simulink model "Roadsense_BehaviourPlanner"  (R2025b)
settings: Solver=FixedStepDiscrete  StartTime=0.0  StopTime=1.0  FixedStep=RsTsBase  RelTol=1e-3
undefined symbols (not defined in the file or in its folder): RsBehaviourEmergencyHoldTicks, RsBehaviourYieldClearTicks, RsGridCols, RsGridRows, RsMaxTracks, RsTsPlanning
settings Model: DataDictionary=Roadsense_Data.sldd  Creator=ragur  LastModifiedBy=ragur

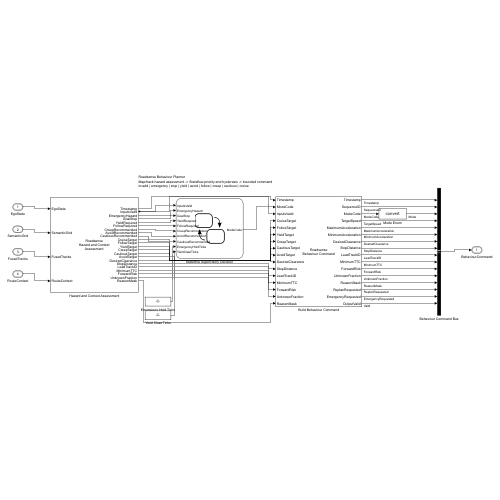
[thumbnail: Simulink's stored preview of the top-level diagram]
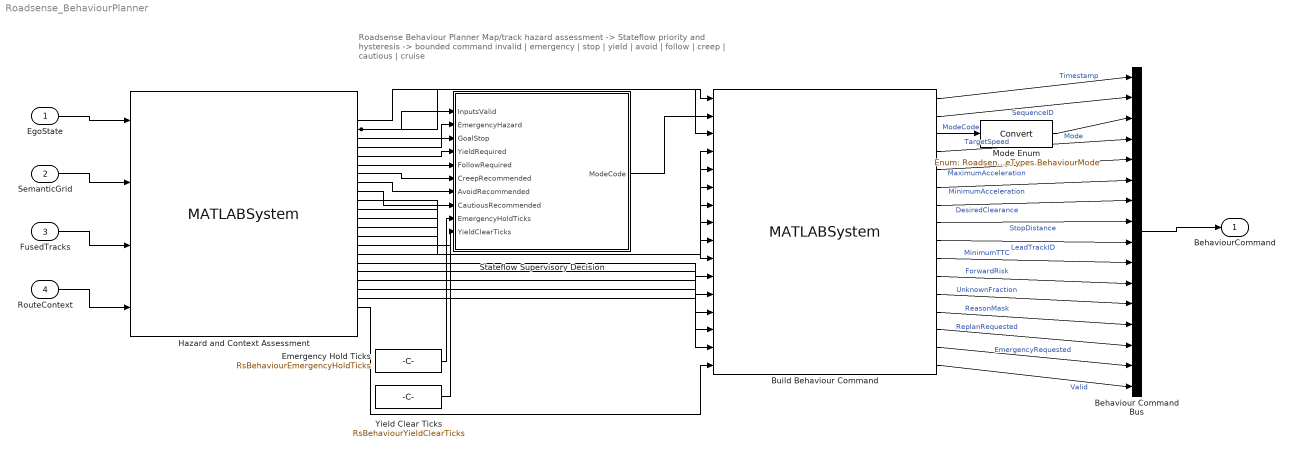
== system Roadsense_BehaviourPlanner ==
  note: Roadsense Behaviour Planner
      | Map/track hazard assessment -> Stateflow priority and hysteresis -> bounded command
      | invalid | emergency | stop | yield | avoid | follow | creep | cautious | cruise
  EgoState : Inport  OutDataTypeStr=Bus: RsEgoStateBus  PortDimensions=1  SampleTime=RsTsPlanning
  SemanticGrid : Inport  Port=2  OutDataTypeStr=Bus: RsSemanticGridBus  PortDimensions=1  SampleTime=RsTsPlanning
  FusedTracks : Inport  Port=3  OutDataTypeStr=Bus: RsFusedTrackListBus  PortDimensions=1  SampleTime=RsTsPlanning
  RouteContext : Inport  Port=4  OutDataTypeStr=Bus: RsRouteContextBus  PortDimensions=1  SampleTime=RsTsPlanning
  Behaviour Command Bus : BusCreator  Inputs=16  OutDataTypeStr=Bus: RsBehaviourCommandBus
  Build Behaviour Command : MATLABSystem  System=RoadsenseBehaviourCommandSystem  SimulateUsing=Code generation
      mask Type: RoadsenseBehaviourCommandSystem
  Emergency Hold Ticks : Constant  Value=RsBehaviourEmergencyHoldTicks  OutDataTypeStr=uint16
  Hazard and Context Assessment : MATLABSystem  System=RoadsenseBehaviourAssessmentSystem  MaxTracks=double(RsMaxTracks)  GridRows=double(RsGridRows)  GridCols=double(RsGridCols)  GridResolution=RsGridResolution  GridXLimits=RsGridXLimits  GridYLimits=RsGridYLimits  ReactionTime=RsBehaviourReactionTime  EmergencyDeceleration=RsBehaviourEmergencyDeceleration  ComfortDeceleration=RsBehaviourComfortDeceleration  EmergencyTTC=RsBehaviourEmergencyTTC  FollowTimeGap=RsBehaviourFollowTimeGap  CreepSpeed=RsBehaviourCreepSpeed  CautiousSpeed=RsBehaviourCautiousSpeed  AvoidSpeed=RsBehaviourAvoidSpeed  SimulateUsing=Code generation
      mask Type: RoadsenseBehaviourAssessmentSystem
  Mode Enum : DataTypeConversion  OutDataTypeStr=Enum: RoadsenseTypes.BehaviourMode  SaturateOnIntegerOverflow=off  RndMeth=Floor
  Stateflow Supervisory Decision : Stateflow chart  TreatAsAtomicUnit=on
  Yield Clear Ticks : Constant  Value=RsBehaviourYieldClearTicks  OutDataTypeStr=uint16
  BehaviourCommand : Outport  OutDataTypeStr=Bus: RsBehaviourCommandBus
  wires:
  EgoState/1 -> Hazard and Context Assessment/1
  SemanticGrid/1 -> Hazard and Context Assessment/2
  FusedTracks/1 -> Hazard and Context Assessment/3
  RouteContext/1 -> Hazard and Context Assessment/4
  Hazard and Context Assessment/2 -> Stateflow Supervisory Decision/1(InputsValid), Build Behaviour Command/3
  Hazard and Context Assessment/3 -> Stateflow Supervisory Decision/2(EmergencyHazard)
  Hazard and Context Assessment/4 -> Stateflow Supervisory Decision/3(GoalStop)
  Hazard and Context Assessment/5 -> Stateflow Supervisory Decision/4(YieldRequired)
  Hazard and Context Assessment/6 -> Stateflow Supervisory Decision/5(FollowRequired)
  Hazard and Context Assessment/7 -> Stateflow Supervisory Decision/6(CreepRecommended)
  Hazard and Context Assessment/8 -> Stateflow Supervisory Decision/7(AvoidRecommended)
  Hazard and Context Assessment/9 -> Stateflow Supervisory Decision/8(CautiousRecommended)
  Emergency Hold Ticks/1 -> Stateflow Supervisory Decision/9(EmergencyHoldTicks)
  Yield Clear Ticks/1 -> Stateflow Supervisory Decision/10(YieldClearTicks)
  Hazard and Context Assessment/1 -> Build Behaviour Command/1
  Stateflow Supervisory Decision/1(ModeCode) -> Build Behaviour Command/2
  Hazard and Context Assessment/10 -> Build Behaviour Command/4
  Hazard and Context Assessment/11 -> Build Behaviour Command/5
  Hazard and Context Assessment/12 -> Build Behaviour Command/6
  Hazard and Context Assessment/13 -> Build Behaviour Command/7
  Hazard and Context Assessment/14 -> Build Behaviour Command/8
  Hazard and Context Assessment/15 -> Build Behaviour Command/9
  Hazard and Context Assessment/16 -> Build Behaviour Command/10
  Hazard and Context Assessment/17 -> Build Behaviour Command/11
  Hazard and Context Assessment/18 -> Build Behaviour Command/12
  Hazard and Context Assessment/19 -> Build Behaviour Command/13
  Hazard and Context Assessment/20 -> Build Behaviour Command/14
  Hazard and Context Assessment/21 -> Build Behaviour Command/15
  Hazard and Context Assessment/22 -> Build Behaviour Command/16
  Build Behaviour Command/3 -> Mode Enum/1  "ModeCode"
  Build Behaviour Command/1 -> Behaviour Command Bus/1  "Timestamp"
  Build Behaviour Command/2 -> Behaviour Command Bus/2  "SequenceID"
  Mode Enum/1 -> Behaviour Command Bus/3  "Mode"
  Build Behaviour Command/4 -> Behaviour Command Bus/4  "TargetSpeed"
  Build Behaviour Command/5 -> Behaviour Command Bus/5  "MaximumAcceleration"
  Build Behaviour Command/6 -> Behaviour Command Bus/6  "MinimumAcceleration"
  Build Behaviour Command/7 -> Behaviour Command Bus/7  "DesiredClearance"
  Build Behaviour Command/8 -> Behaviour Command Bus/8  "StopDistance"
  Build Behaviour Command/9 -> Behaviour Command Bus/9  "LeadTrackID"
  Build Behaviour Command/10 -> Behaviour Command Bus/10  "MinimumTTC"
  Build Behaviour Command/11 -> Behaviour Command Bus/11  "ForwardRisk"
  Build Behaviour Command/12 -> Behaviour Command Bus/12  "UnknownFraction"
  Build Behaviour Command/13 -> Behaviour Command Bus/13  "ReasonMask"
  Build Behaviour Command/14 -> Behaviour Command Bus/14  "ReplanRequested"
  Build Behaviour Command/15 -> Behaviour Command Bus/15  "EmergencyRequested"
  Build Behaviour Command/16 -> Behaviour Command Bus/16  "Valid"
  Behaviour Command Bus/1 -> BehaviourCommand/1

== stateflow chart Roadsense_BehaviourPlanner/Stateflow Supervisory Decision ==
  state SupervisoryDecision
    entry:
    PreviousMode = uint8(0);
    EmergencyHoldCounter = uint16(0);
    YieldClearCounter = uint16(0);
    ModeCode = uint8(0);
    during:
    [ModeCode, EmergencyHoldCounter, YieldClearCounter] = ...
    RoadsenseBehaviourDecisionCore(InputsValid, EmergencyHazard, GoalStop, ...
    YieldRequired, FollowRequired, CreepRecommended, AvoidRecommended, ...
    CautiousRecommended, PreviousMode, EmergencyHoldCounter, ...
    YieldClearCounter, EmergencyHoldTicks, YieldClearTicks);
    PreviousMode = ModeCode;
  (default) -> SupervisoryDecision
  data: InputsValid input boolean; EmergencyHazard input boolean; GoalStop input boolean; YieldRequired input boolean; FollowRequired input boolean; CreepRecommended input boolean; AvoidRecommended input boolean; CautiousRecommended input boolean; EmergencyHoldTicks input uint16; YieldClearTicks input uint16; ModeCode output uint8; PreviousMode local uint8; EmergencyHoldCounter local uint16; YieldClearCounter local uint16
